simulink model "BuildFlexionExtension2024a"  (R2024a)
settings: Solver=FixedStepAuto  StartTime=0.0  StopTime=inf  FixedStep=1/100  RelTol=1e-3
InitFcn:
  | bp= [0 1 2  5  7  12 16 20 24 28 32 36 40 42 44 46 48 50];
  | spl=[0 3 8 15  25 34 45 60 76 96 110 120 130 138 145 150 155 158]/158;
  | 
  | breakp=[-fliplr(bp(2:end)) bp]*pi/180;
  | spline=[-fliplr(spl(2:end)) spl];
undefined symbols (not defined in the file): Discrete, FSset, Low, qbreak, Time
libraries: arduinolib x34, dspswit3 x11, etargetslib x8, canmsglib x5, dspfdesign x2, ctrlSharedLib x1
settings Model: SimulationMode=external  ExtModeTrigDuration=2  Creator=alexx  LastModifiedBy=roman
settings SolverCC: AutoInsertRateTranBlk=on
settings OptimizationCC: EnhancedBackFolding=on  PassReuseOutputArgsAs=Individual arguments  ZeroExternalMemoryAtStartup=off  ZeroInternalMemoryAtStartup=off  MaxStackSize=64  OptimizeBlockOrder=speed  DifferentSizesBufferReuse=on  OptimizationCustomize=off  EfficientTunableParamExpr=on
settings DebuggingCC: MultiTaskCondExecSysMsg=none  ParameterTunabilityLossMsg=error
settings HardwareCC: ProdBitPerPointer=32  ProdBitPerSizeT=32  ProdBitPerPtrDiffT=32  ProdLargestAtomicInteger=Long  ProdLargestAtomicFloat=Double  ProdWordSize=32  ProdHWDeviceType=ARM Compatible->ARM Cortex  UseEmbeddedCoderFeatures=off  UseSimulinkCoderFeatures=off
settings SFSimCC: MATLABDynamicMemAlloc=off
settings RTWCC: Description=Embedded Coder  SystemTargetFile=ert.tlc  HardwareBoard=Arduino MKR WiFi 1010  TemplateMakefile=ert_default_tmf  Toolchain=Arduino ARM  BuildConfiguration=Faster Runs  GPUComputeCapability=3.5
settings CodeAppCC: ForceParamTrailComments=on  IgnoreCustomStorageClasses=off  OperatorAnnotations=on  SimulinkDataObjDesc=on  SFDataObjDesc=on  InsertBlockDesc=on
settings ERTTargetCC: SupportContinuousTime=on  SupportNonInlinedSFcns=on  SupportVariableSizeSignals=on  ExtModeTransport=3  ExtModeStaticAlloc=on  ExtModeAutomaticAllocSize=off  ExtModeStaticAllocSize=8192  ExtModeMexFile=ext_xcp  ExtModeIntrfLevel=Level2 - Open
settings ConfigComp: CovBoundaryAbsTol=1.0e-5

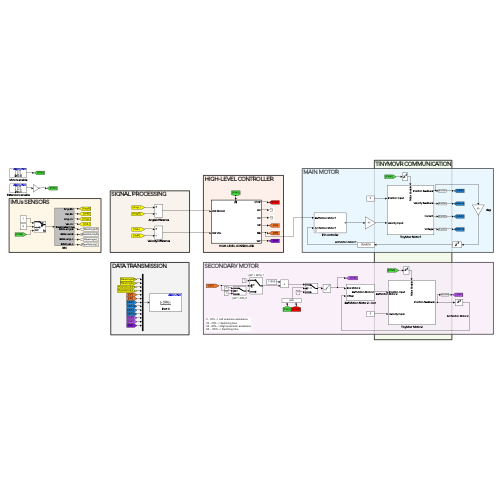
[thumbnail: Simulink's stored preview of the top-level diagram]
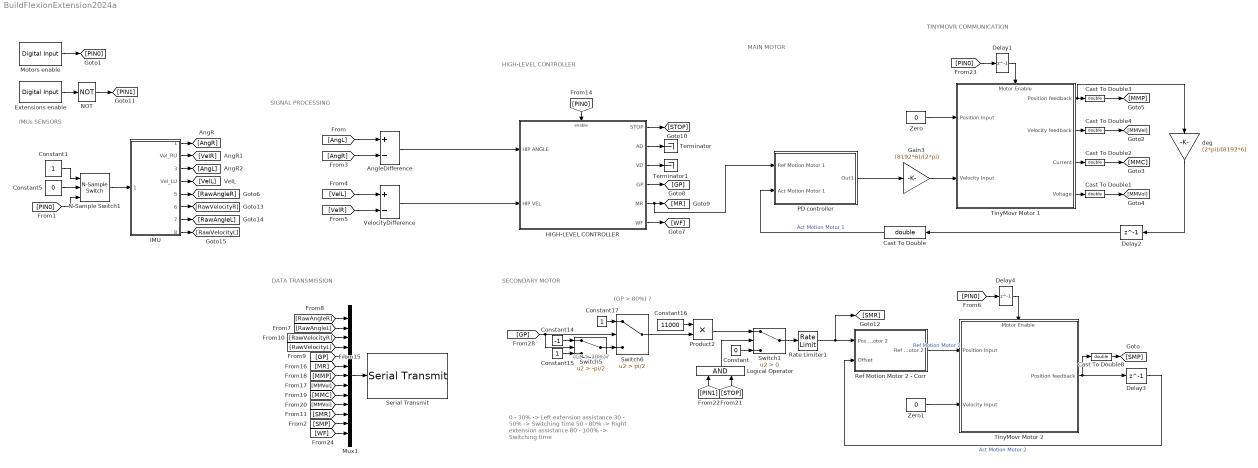
== system BuildFlexionExtension2024a ==
  note: 0 - 30% -> Left extension assistance
      | 30 - 50% -> Switching time
      | 50 - 80% -> Right extension assistance
      | 80 - 100% -> Switching time
  note: (GP > 30%)?
  note: DATA TRANSMISSION
  note: TINYMOVR COMMUNICATION
  note: MAIN MOTOR
  note: SECONDARY MOTOR
  note: HIGH-LEVEL CONTROLLER
  note: SIGNAL PROCESSING
  note: IMUs SENSORS
  note: (GP > 80%) ?
  AngleDifference : Sum  Inputs=+-
  Cast To Double{,1..4,8} (6 alike) : DataTypeConversion  OutDataTypeStr=double  SaturateOnIntegerOverflow=off  RndMeth=Floor
  Constant : Constant  Value=0
  Constant1 : Constant
  Constant14 : Constant  Value=-1
  Constant15 : Constant
  Constant16 : Constant  Value=11000
  Constant17 : Constant
  Constant5 : Constant  Value=0
  Delay{1..4} (4 alike) : Delay  DelayLength=1
  Extensions enable : arduinolib/Digital Input  pinNumber=1  mode=Input Pullup  Direction=input  SampleTime=1/100  blockPlatform=arduino
  Gain3 : Gain  Gain=(8192*6)/(2*pi)  ParamDataTypeStr=single  OutDataTypeStr=single
  HIGH-LEVEL CONTROLLER : Subsystem
  IMU : Subsystem
  Logical Operator : Logic  AllPortsSameDT=off  OutDataTypeStr=boolean
  Motors enable : arduinolib/Digital Input  pinNumber=0  mode=Default  Direction=input  SampleTime=1/100  blockPlatform=arduino
  Mux1 : Mux  Inputs=13
  N-Sample Switch1 : dspswit3/N-Sample Switch  N=10  reset=on  TriggerType=Rising edge  Ts=-1
  NOT : Logic  Operator=NOT  IconShape=distinctive  AllPortsSameDT=off  OutDataTypeStr=boolean
  PD controller : Subsystem  mask{Kp=12, Ki=0, Kd=0.2}
      mask prompts: Kp "P"; Ki "I"; Kd "D"
      mask DialogControl DescGroupVar Prompt: PID Parameters
      mask DialogControl DescTextVar Prompt: Select the values for P I D parameters
  Product2 : Product
  Rate Limiter1 : RateLimiter  RisingSlewLimit=480000  FallingSlewLimit=-480000
  Ref Motion Motor 2 - Corr : Subsystem
  Serial Transmit : arduinolib/Serial Transmit  portNumber=0  sendmode=write  sendformat=Decimal  floatprecision=2  header=[]  terminator=[]  blockPlatform=ARDUINO
  Switch1 : Switch  Criteria=u2 > Threshold  SaturateOnIntegerOverflow=off  InputSameDT=off
  Switch5 : Switch  Criteria=u2 > Threshold  Threshold=-pi/2  SaturateOnIntegerOverflow=off  InputSameDT=off
  Switch6 : Switch  Criteria=u2 > Threshold  Threshold=pi/2  SaturateOnIntegerOverflow=off  InputSameDT=off
  Terminator : Terminator
  Terminator1 : Terminator
  TinyMovr Motor 1 : Subsystem
      settings: PortSchema="{\"entries\":[{\"content\":{\"sides\":[{\"content\":{\"connectorIds\":[\"In1\",\"In2\"]},\"type\":\"ConnectorPlacement.EquallySpacedRectSide\",\"uuid\":\"96eb0664-e7f9-4da5-900f-02ca39bdcd94\"},{\"content\":{\"connectorIds\":[\"Out1\",\"Out2\",\"Out3\",\"Out4\"],\"side\":\"RIGHT\"},\"type\":\"ConnectorPlacement.EquallySpacedRectSide\",\"uuid\":\"3b096aff-b574-48d5-b85c-bddb8debe324\"},{\"content\":{\"connectorIds\":[\"In3\"],\"side\":\"TOP\"},\"type\":\"ConnectorPlacement.EquallySpacedRectSide\",\"uuid\":\"4d311d4a-d713-49d1-a682-ce685fb67b1a\"},{\"content\":{\"side\":\"BOTTOM\"},\"type\":\"ConnectorPlacement.EquallySpacedRectSide\",\"uuid\":\"60a29e50-835b-4a88-8a5f-1647b9a36173\"}]},\"type\":\"ConnectorPlacement.EquallySpacedConnector\",\"uuid\":\"850c9b35-9cb9-4fb8-b21d-22107ea3627a\"}],\"packageUris\":[\"http://schema.mathworks.com/mf0/Connector/R2020b\"],\"version\":\"1.0\"}"
  TinyMovr Motor 2 : Subsystem
      settings: PortSchema="{\"entries\":[{\"content\":{\"sides\":[{\"content\":{\"connectorIds\":[\"In1\",\"In2\"]},\"type\":\"ConnectorPlacement.EquallySpacedRectSide\",\"uuid\":\"96eb0664-e7f9-4da5-900f-02ca39bdcd94\"},{\"content\":{\"connectorIds\":[\"Out1\"],\"side\":\"RIGHT\"},\"type\":\"ConnectorPlacement.EquallySpacedRectSide\",\"uuid\":\"3b096aff-b574-48d5-b85c-bddb8debe324\"},{\"content\":{\"connectorIds\":[\"In3\"],\"side\":\"TOP\"},\"type\":\"ConnectorPlacement.EquallySpacedRectSide\",\"uuid\":\"4d311d4a-d713-49d1-a682-ce685fb67b1a\"}]},\"type\":\"ConnectorPlacement.EquallySpacedConnector\",\"uuid\":\"850c9b35-9cb9-4fb8-b21d-22107ea3627a\"}],\"packageUris\":[\"http://schema.mathworks.com/mf0/Connector/R2020b\"],\"version\":\"1.0\"}"
  VelocityDifference : Sum  Inputs=+-
  Zero : Constant  Value=0  OutDataTypeStr=single
  Zero1 : Constant  Value=0  OutDataTypeStr=single
  deg : Gain  Gain=(2*pi)/(8192*6)  ParamDataTypeStr=single  OutDataTypeStr=single
  wires:
  Cast To Double/1 -> PD controller/2(Act Motion Motor 1)  "Act Motion Motor 1"
  Delay3/1 -> Ref Motion Motor 2 - Corr/2(Offset)  "Act Motion Motor 2"
  TinyMovr Motor 1/1(Position feedback) -> deg/1, Cast To Double3/1
  Ref Motion Motor 2 - Corr/1(Ref Motion Motor 2) -> TinyMovr Motor 2/1(Position Input)  "Ref Motion Motor 2"
  Delay1/1 -> TinyMovr Motor 1/3(Motor Enable)
  Zero/1 -> TinyMovr Motor 1/1(Position Input)
  PD controller/1(Out1) -> Gain3/1
  deg/1 -> Delay2/1
  TinyMovr Motor 2/1(Position feedback) -> Delay3/1, Cast To Double8/1
  Gain3/1 -> TinyMovr Motor 1/2(Velocity Input)
  Rate Limiter1/1 -> Ref Motion Motor 2 - Corr/1(Pos Motor 2), [SMR]
  N-Sample Switch1/1 -> IMU/1(BaselineRemove)
  Constant5/1 -> N-Sample Switch1/2
  Constant1/1 -> N-Sample Switch1/1
  [PIN0] -> N-Sample Switch1/3
  [PIN0] -> HIGH-LEVEL CONTROLLER/Enable
  [PIN0] -> Delay1/1
  HIGH-LEVEL CONTROLLER/5(MR) -> PD controller/1(Ref Motion Motor 1), [MR]
  HIGH-LEVEL CONTROLLER/1(STOP) -> [STOP]
  AngleDifference/1 -> HIGH-LEVEL CONTROLLER/1(HIP ANGLE)
  VelocityDifference/1 -> HIGH-LEVEL CONTROLLER/2(HIP VEL)
  Mux1/1 -> Serial Transmit/1
  [AngL] -> AngleDifference/1
  [AngR] -> AngleDifference/2
  [VelL] -> VelocityDifference/1
  [VelR] -> VelocityDifference/2
  Delay2/1 -> Cast To Double/1
  Zero1/1 -> TinyMovr Motor 2/2(Velocity Input)
  [PIN0] -> Delay4/1
  Delay4/1 -> TinyMovr Motor 2/3(Motor Enable)
  IMU/1(Ang_RU) -> [AngR]
  IMU/2(Vel_RU) -> [VelR]
  IMU/3(Ang_LU) -> [AngL]
  IMU/4(Vel_LU) -> [VelL]
  [RawAngleR] -> Mux1/1
  [RawAngleL] -> Mux1/2
  [RawVelocityR] -> Mux1/3
  [RawVelocityL] -> Mux1/4
  TinyMovr Motor 1/2(Velocity feedback) -> Cast To Double4/1
  TinyMovr Motor 1/3(Current) -> Cast To Double2/1
  TinyMovr Motor 1/4(Voltage) -> Cast To Double1/1
  Cast To Double8/1 -> [SMP]
  [GP] -> Mux1/5
  [MR] -> Mux1/6
  [MMP] -> Mux1/7
  [MMVel] -> Mux1/8
  [MMC] -> Mux1/9
  [MMVol] -> Mux1/10
  Cast To Double1/1 -> [MMVol]
  Cast To Double2/1 -> [MMC]
  Cast To Double4/1 -> [MMVel]
  Cast To Double3/1 -> [MMP]
  HIGH-LEVEL CONTROLLER/2(AD) -> Terminator/1
  HIGH-LEVEL CONTROLLER/3(VD) -> Terminator1/1
  HIGH-LEVEL CONTROLLER/4(GP) -> [GP]
  [STOP] -> Logical Operator/2
  Switch1/1 -> Rate Limiter1/1
  Extensions enable/1 -> NOT/1
  Logical Operator/1 -> Switch1/2
  [PIN1] -> Logical Operator/1
  Constant/1 -> Switch1/3
  NOT/1 -> [PIN1]
  Motors enable/1 -> [PIN0]
  [SMP] -> Mux1/12
  [SMR] -> Mux1/11
  [GP] -> Switch6/2, Switch5/2
  Constant14/1 -> Switch5/1
  Constant15/1 -> Switch5/3
  Constant17/1 -> Switch6/1
  Switch5/1 -> Switch6/3
  Product2/1 -> Switch1/1
  Constant16/1 -> Product2/1
  Switch6/1 -> Product2/2
  HIGH-LEVEL CONTROLLER/6(WF) -> [WF]
  [WF] -> Mux1/13
  IMU/5(RAW_ang_R) -> [RawAngleR]
  IMU/6(RAW_vel_R) -> [RawVelocityR]
  IMU/7(RAW_ang_L) -> [RawAngleL]
  IMU/8(RAW_vel_L) -> [RawVelocityL]

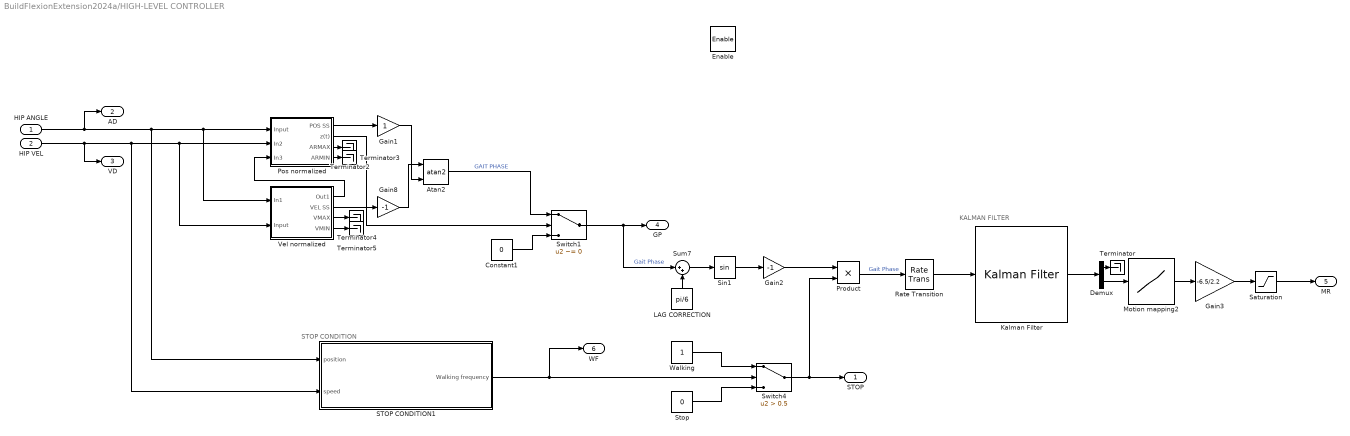
== system BuildFlexionExtension2024a/HIGH-LEVEL CONTROLLER ==
  note: KALMAN FILTER
  note: STOP CONDITION
  HIP ANGLE : Inport
  HIP VEL : Inport  Port=2
  Enable : EnablePort  StatesWhenEnabling=reset
  Atan2 : Trigonometry  Operator=atan2
  Constant1 : Constant  Value=0
  Demux : Demux  Outputs=2
  Gain1 : Gain
  Gain2 : Gain  Gain=-1
  Gain3 : Gain  Gain=-6.5/2.2
  Gain8 : Gain  Gain=-1
  Kalman Filter : ctrlSharedLib/Kalman Filter  TimeDomain=Discrete-Time  UseCurrentEstimator=on  ModelSource=Individual A, B, C, D matrices  ModelSourceVariable=idss  A=[1 0.01;0 1]  B=eye(2)  C=[1 0]  D=zeros(2)  NumberOfStates=1  NumberOfInputs=1  NumberOfOutputs=1  InitialEstimateSource=Dialog  X0=0  P0=10  UseK=off  UseGH=off  NumberOfProcessNoiseInputs=2  G=1  TimeInvariantG=on  H=0  TimeInvariantH=on  Q=0.02  TimeInvariantQ=on  R=0.75  TimeInvariantR=on  N=0  TimeInvariantN=on  AddInputPort=off  AddEnablePort=off  OutputEstimatedY=off  OutputP=off  Ts=-1
  LAG CORRECTION : Constant  Value=pi/6
  Motion mapping2 : Lookup_n-D  NumberOfTableDimensions=1  BreakpointsForDimension1=breakp  BreakpointsForDimension2=qbreak(:,2)  Table=spline  InterpMethod=Cubic spline  ExtrapMethod=Cubic spline  InternalRulePriority=Speed  RndMeth=Simplest
  Pos normalized : Subsystem
  Product : Product
  Rate Transition : RateTransition  OutPortSampleTime=0.01
  STOP CONDITION1 : Subsystem
  Saturation : Saturate  UpperLimit=600*pi/180  LowerLimit=-600*pi/180
  Sin1 : Trigonometry
  Stop : Constant  Value=0
  Sum7 : Sum  Inputs=|++
  Switch1 : Switch  Criteria=u2 ~= 0  SaturateOnIntegerOverflow=off  InputSameDT=off
  Switch4 : Switch  Criteria=u2 > Threshold  Threshold=0.5  SaturateOnIntegerOverflow=off  InputSameDT=off
  Terminator{,2..5} (5 alike) : Terminator
  Vel normalized : Subsystem
  Walking : Constant
  STOP : Outport
  AD : Outport  Port=2
  VD : Outport  Port=3
  GP : Outport  Port=4
  MR : Outport  Port=5
  WF : Outport  Port=6
  wires:
  Kalman Filter/1 -> Demux/1
  Gain8/1 -> Atan2/1
  Gain2/1 -> Product/1
  Gain3/1 -> Saturation/1
  Rate Transition/1 -> Kalman Filter/1
  Atan2/1 -> Switch1/1  "GAIT PHASE"
  Sin1/1 -> Gain2/1
  Switch1/1 -> GP/1, Sum7/1  "Gait Phase"
  Product/1 -> Rate Transition/1  "Gait Phase"
  Constant1/1 -> Switch1/3
  Motion mapping2/1 -> Gain3/1
  Demux/1 -> Terminator/1
  LAG CORRECTION/1 -> Sum7/2
  Gain1/1 -> Atan2/2
  Saturation/1 -> MR/1
  Pos normalized/1(POS SS) -> Gain1/1
  Pos normalized/2(z(t)) -> Switch1/2
  Vel normalized/1(Out1) -> Pos normalized/3(In3)
  Vel normalized/2(VEL SS) -> Gain8/1
  Pos normalized/3(ARMAX) -> Terminator2/1
  Pos normalized/4(ARMIN) -> Terminator3/1
  Vel normalized/3(VMAX) -> Terminator4/1
  Vel normalized/4(VMIN) -> Terminator5/1
  Sum7/1 -> Sin1/1
  Demux/2 -> Motion mapping2/1
  Walking/1 -> Switch4/1
  HIP VEL/1 -> VD/1, STOP CONDITION1/2(speed), Vel normalized/2(Input), Pos normalized/2(In2)
  Switch4/1 -> STOP/1, Product/2
  Stop/1 -> Switch4/3
  STOP CONDITION1/1(Walking frequency) -> WF/1, Switch4/2
  HIP ANGLE/1 -> STOP CONDITION1/1(position), Vel normalized/1(In1), Pos normalized/1(Input), AD/1

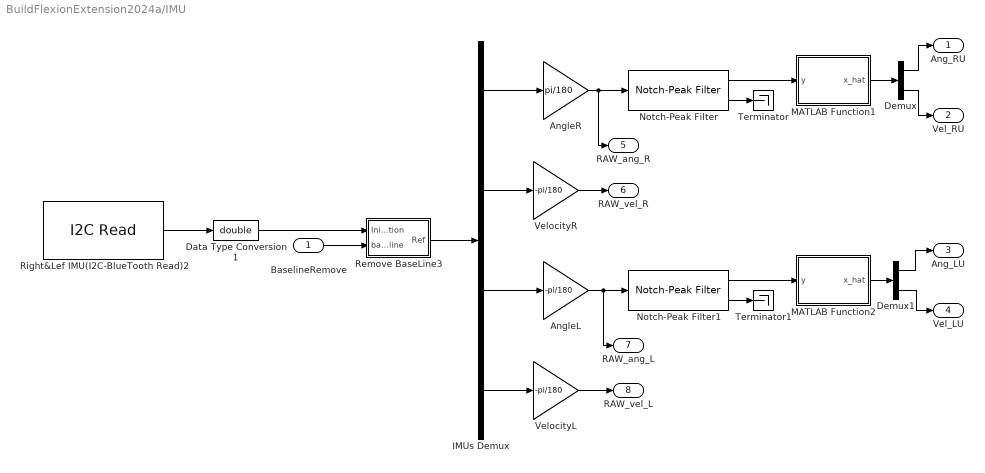
== system BuildFlexionExtension2024a/IMU ==
  BaselineRemove : Inport
  AngleL : Gain  Gain=-pi/180
  AngleR : Gain  Gain=pi/180
  Data Type Conversion1 : DataTypeConversion  OutDataTypeStr=double  SaturateOnIntegerOverflow=off  RndMeth=Floor
  Demux : Demux  Outputs=2
  Demux1 : Demux  Outputs=2
  IMUs Demux : Demux
  MATLAB Function1 : MATLAB Function  TreatAsAtomicUnit=on
  MATLAB Function2 : MATLAB Function  TreatAsAtomicUnit=on
  Notch-Peak Filter : dspfdesign/Notch-Peak Filter  Specification=Bandwidth and center frequency  BandwidthPort=off  Bandwidth=0.1  QualityFactorPort=off  QualityFactor=5  CenterFrequencyPort=off  CenterFrequency=0  BandwidthCoefficientPort=off  BandwidthCoefficient=0.72654  CenterFrequencyCoefficientPort=off  CenterFrequencyCoefficient=0  Output=Notch and Peak  SampleRateMode=Specify on dialog  SampleRate=100  SimulateUsing=Code generation
  Notch-Peak Filter1 : dspfdesign/Notch-Peak Filter  Specification=Bandwidth and center frequency  BandwidthPort=off  Bandwidth=0.1  QualityFactorPort=off  QualityFactor=5  CenterFrequencyPort=off  CenterFrequency=0  BandwidthCoefficientPort=off  BandwidthCoefficient=0.72654  CenterFrequencyCoefficientPort=off  CenterFrequencyCoefficient=0  Output=Notch and Peak  SampleRateMode=Specify on dialog  SampleRate=100  SimulateUsing=Code generation
  Remove BaseLine3 : Subsystem
  Right&Lef IMU(I2C-BlueTooth Read)2 : arduinolib/I2C Read  I2CModule=0  Mode=Master  SlaveAddress=45  SlaveByteOrder=LittleEndian  Direction=Receiver  RegisterAddressMode=off  RegisterAddress=0  SlaveDataType=single  DataLength=4  NoAck=off  RepeatedStart=off  OutputStatus=off  blockPlatform=ARDUINO  SampleTime=0.01
  Terminator : Terminator
  Terminator1 : Terminator
  VelocityL : Gain  Gain=-pi/180
  VelocityR : Gain  Gain=-pi/180
  Ang_RU : Outport
  Vel_RU : Outport  Port=2
  Ang_LU : Outport  Port=3
  Vel_LU : Outport  Port=4
  RAW_ang_R : Outport  Port=5
  RAW_vel_R : Outport  Port=6
  RAW_ang_L : Outport  Port=7
  RAW_vel_L : Outport  Port=8
  wires:
  BaselineRemove/1 -> Remove BaseLine3/2(baseline)
  Data Type Conversion1/1 -> Remove BaseLine3/1(Initial Motion)
  Right&Lef IMU(I2C-BlueTooth Read)2/1 -> Data Type Conversion1/1
  Remove BaseLine3/1(Ref) -> IMUs Demux/1
  IMUs Demux/2 -> VelocityR/1
  IMUs Demux/1 -> AngleR/1
  AngleR/1 -> RAW_ang_R/1, Notch-Peak Filter/1
  IMUs Demux/3 -> AngleL/1
  IMUs Demux/4 -> VelocityL/1
  AngleL/1 -> RAW_ang_L/1, Notch-Peak Filter1/1
  Notch-Peak Filter/1 -> MATLAB Function1/1(y)
  Notch-Peak Filter/2 -> Terminator/1
  Notch-Peak Filter1/1 -> MATLAB Function2/1(y)
  Notch-Peak Filter1/2 -> Terminator1/1
  MATLAB Function1/1(x_hat) -> Demux/1
  Demux/1 -> Ang_RU/1
  Demux/2 -> Vel_RU/1
  MATLAB Function2/1(x_hat) -> Demux1/1
  Demux1/1 -> Ang_LU/1
  Demux1/2 -> Vel_LU/1
  VelocityR/1 -> RAW_vel_R/1
  VelocityL/1 -> RAW_vel_L/1

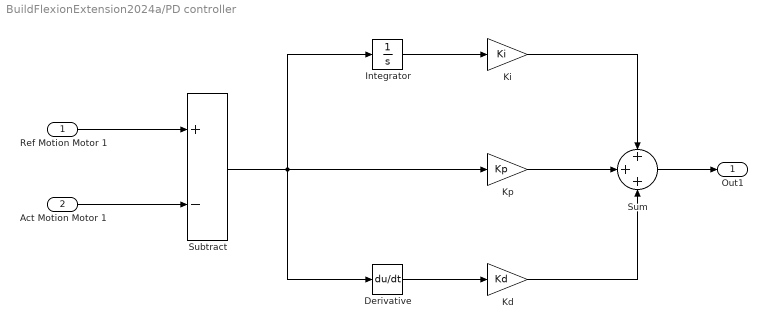
== system BuildFlexionExtension2024a/PD controller ==
  Ref Motion Motor 1 : Inport
  Act Motion Motor 1 : Inport  Port=2
  Derivative : Derivative
  Integrator : Integrator
  Kd : Gain  Gain=Kd
  Ki : Gain  Gain=Ki
  Kp : Gain  Gain=Kp
  Subtract : Sum  Inputs=+-
  Sum : Sum  Inputs=+++
  Out1 : Outport
  wires:
  Act Motion Motor 1/1 -> Subtract/2
  Ref Motion Motor 1/1 -> Subtract/1
  Integrator/1 -> Ki/1
  Sum/1 -> Out1/1
  Ki/1 -> Sum/1
  Kp/1 -> Sum/2
  Kd/1 -> Sum/3
  Subtract/1 -> Derivative/1, Kp/1, Integrator/1
  Derivative/1 -> Kd/1

== system BuildFlexionExtension2024a/Ref Motion Motor 2 - Corr ==
  note: The blocks are making sure the motor’s commanded motion is always consistent with its measured position. If the encoder hasn’t moved (maybe at power-up or during a pause), the system falls back to an offset value. The sum block then adjusts the commanded trajectory by this alignment term, so the reference sent to the motor matches reality.
  Pos Motor 2 : Inport
  Offset : Inport  Port=2
  Add : Sum
  Constant : Constant  Value=0
  Delay : Delay  DelayLength=1
  Delay1 : Delay  DelayLength=1
  Switch1 : Switch  Criteria=u2 ~= 0  SaturateOnIntegerOverflow=off  InputSameDT=off
  Ref Motion Motor 2 : Outport
  wires:
  Offset/1 -> Delay1/1  "Motor Encoder [rad]"
  Delay1/1 -> Switch1/2
  Switch1/1 -> Delay/1, Add/2
  Delay/1 -> Switch1/1
  Add/1 -> Ref Motion Motor 2/1
  Pos Motor 2/1 -> Add/1
  Constant/1 -> Switch1/3

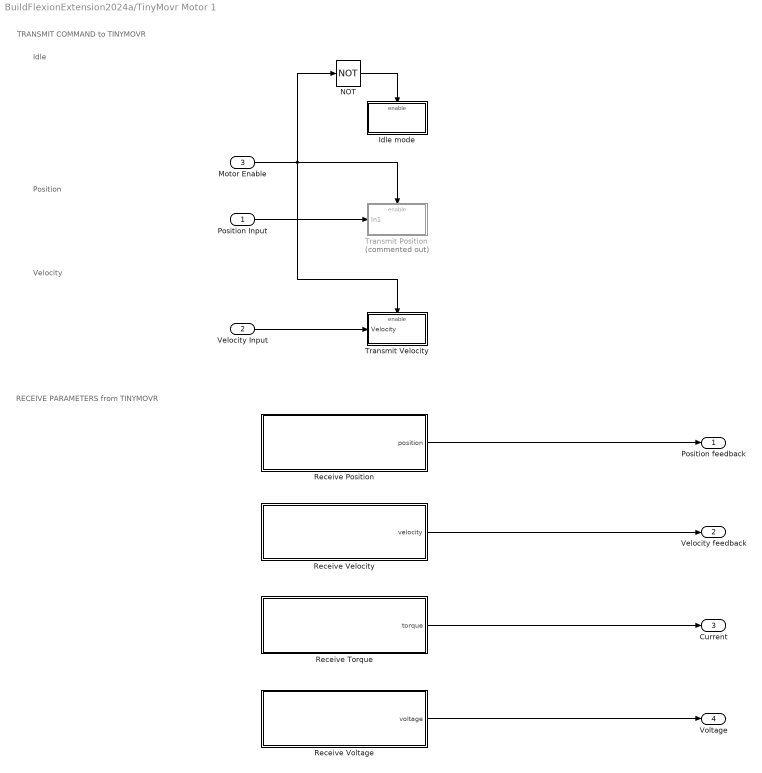
== system BuildFlexionExtension2024a/TinyMovr Motor 1 ==
  note: Idle
  note: Velocity
  note: TRANSMIT COMMAND to TINYMOVR
  note: Position
  note: RECEIVE PARAMETERS from TINYMOVR
  Position Input : Inport
  Velocity Input : Inport  Port=2
  Motor Enable : Inport  Port=3
  Idle mode : Subsystem  TreatAsAtomicUnit=on
  NOT : Logic  Operator=NOT  AllPortsSameDT=off  OutDataTypeStr=boolean
  Receive Position : Subsystem
  Receive Torque : Subsystem
  Receive Velocity : Subsystem
  Receive Voltage : Subsystem
  Transmit Position : Subsystem  Commented=on  TreatAsAtomicUnit=on
  Transmit Velocity : Subsystem  TreatAsAtomicUnit=on
  Position feedback : Outport
  Velocity feedback : Outport  Port=2
  Current : Outport  Port=3
  Voltage : Outport  Port=4
  wires:
  Position Input/1 -> Transmit Position/1(In1)
  NOT/1 -> Idle mode/Enable
  Motor Enable/1 -> Transmit Position/Enable, Transmit Velocity/Enable, NOT/1
  Velocity Input/1 -> Transmit Velocity/1(Velocity)
  Receive Position/1(position) -> Position feedback/1
  Receive Velocity/1(velocity) -> Velocity feedback/1
  Receive Torque/1(torque) -> Current/1
  Receive Voltage/1(voltage) -> Voltage/1

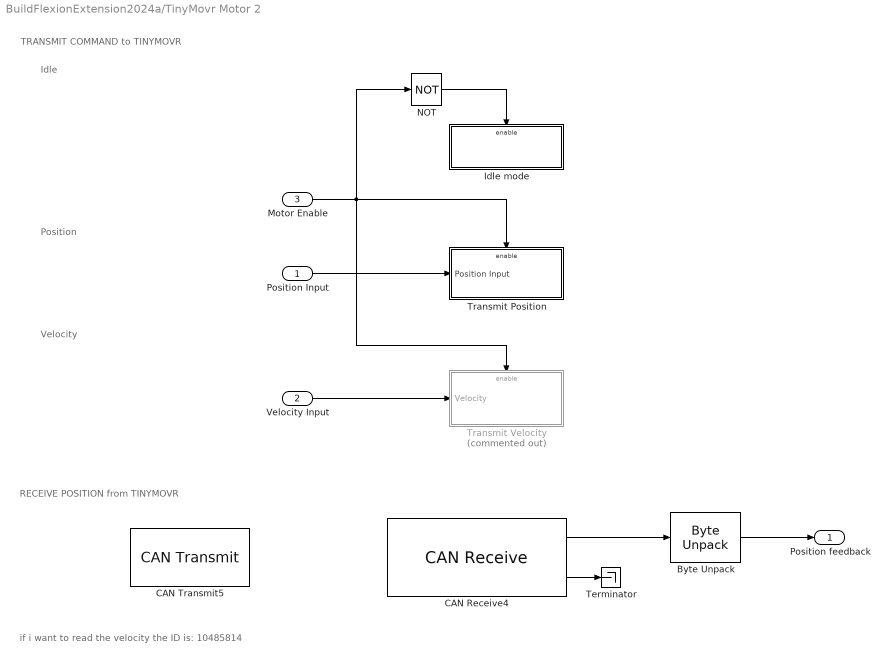
== system BuildFlexionExtension2024a/TinyMovr Motor 2 ==
  note: if i want to read the velocity the ID is: 10485814
  note: Idle
  note: Velocity
  note: TRANSMIT COMMAND to TINYMOVR
  note: RECEIVE POSITION from TINYMOVR
  note: Position
  Position Input : Inport
  Velocity Input : Inport  Port=2
  Motor Enable : Inport  Port=3
  Byte Unpack : etargetslib/Byte Unpack  dimensions={[1]}  datatypes={'single'}  byteAlign=1
      settings: LibrarySourceBlock=embeddedtargetslib/Host Communication/Byte Unpack
  CAN Receive4 : arduinolib/CAN Receive  outputDataType=Raw data  identifierType=Extended (29-bit identifier)  messageId=4194359  msgLength=4  SampleTime=0.01  outputError=off  outputRemote=off
  CAN Transmit5 : arduinolib/CAN Transmit  inputDataType=Raw data  BlockingMode_=off  BlockTimeout_=1  outputStatus=off  identifierType=Extended (29-bit identifier)  messageId=4194359  msgLength=0  remoteFrame=on
  Idle mode : Subsystem  TreatAsAtomicUnit=on
  NOT : Logic  Operator=NOT  AllPortsSameDT=off  OutDataTypeStr=boolean
  Terminator : Terminator
  Transmit Position : Subsystem  TreatAsAtomicUnit=on
  Transmit Velocity : Subsystem  Commented=on  TreatAsAtomicUnit=on
  Position feedback : Outport
  wires:
  CAN Receive4/1 -> Byte Unpack/1
  CAN Receive4/2 -> Terminator/1
  Byte Unpack/1 -> Position feedback/1
  Position Input/1 -> Transmit Position/1(Position Input)
  NOT/1 -> Idle mode/Enable
  Velocity Input/1 -> Transmit Velocity/1(Velocity)
  Motor Enable/1 -> Transmit Position/Enable, Transmit Velocity/Enable, NOT/1

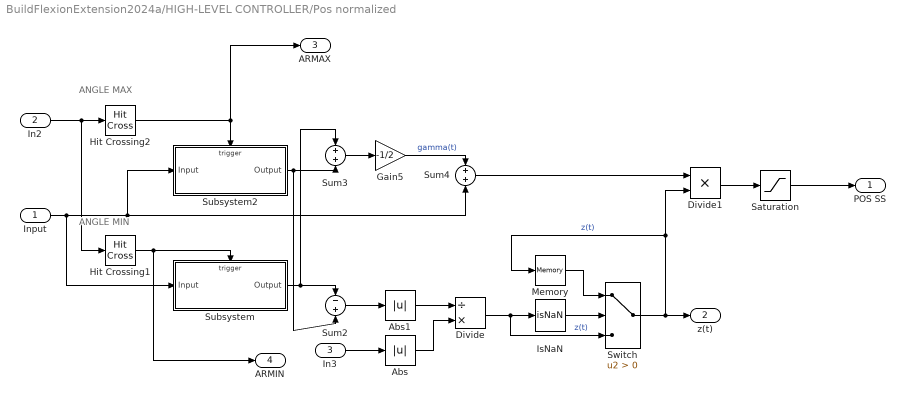
== system BuildFlexionExtension2024a/HIGH-LEVEL CONTROLLER/Pos normalized ==
  note: ANGLE MIN
  note: ANGLE MAX
  Input : Inport
  In2 : Inport  Port=2
  In3 : Inport  Port=3
  Abs : Abs  SaturateOnIntegerOverflow=off
  Abs1 : Abs  SaturateOnIntegerOverflow=off
  Divide : Product  Inputs=/*
  Divide1 : Product  Inputs=**
  Gain5 : Gain  Gain=-1/2
  Hit Crossing1 : HitCross  HitCrossingOffset=-1  HitCrossingDirection=rising
  Hit Crossing2 : HitCross  HitCrossingOffset=1  HitCrossingDirection=falling
  IsNaN : RelationalOperator  Operator=isNaN  OutDataTypeStr=boolean  RndMeth=Simplest  InputSameDT=off
  Memory : Memory
  Saturation : Saturate  UpperLimit=10  LowerLimit=-10
  Subsystem : Subsystem
  Subsystem2 : Subsystem
  Sum2 : Sum  Inputs=-+
  Sum3 : Sum
  Sum4 : Sum
  Switch : Switch  Criteria=u2 > Threshold  SaturateOnIntegerOverflow=off  InputSameDT=off
  POS SS : Outport
  z(t) : Outport  Port=2
  ARMAX : Outport  Port=3
  ARMIN : Outport  Port=4
  wires:
  Hit Crossing2/1 -> Subsystem2/Trigger, ARMAX/1
  Subsystem2/1(Output) -> Sum3/2, Sum2/2
  Sum4/1 -> Divide1/1
  Sum3/1 -> Gain5/1
  Subsystem/1(Output) -> Sum2/1, Sum3/1
  Hit Crossing1/1 -> ARMIN/1, Subsystem/Trigger
  Input/1 -> Subsystem2/1(Input), Sum4/2, Subsystem/1(Input)
  In2/1 -> Hit Crossing1/1, Hit Crossing2/1
  Sum2/1 -> Abs1/1
  In3/1 -> Abs/1
  Gain5/1 -> Sum4/1  "gamma(t)"
  Abs1/1 -> Divide/1
  Abs/1 -> Divide/2
  Divide/1 -> IsNaN/1, Switch/3  "z(t)"
  Memory/1 -> Switch/1
  IsNaN/1 -> Switch/2
  Switch/1 -> Memory/1, Divide1/2, z(t)/1  "z(t)"
  Divide1/1 -> Saturation/1
  Saturation/1 -> POS SS/1

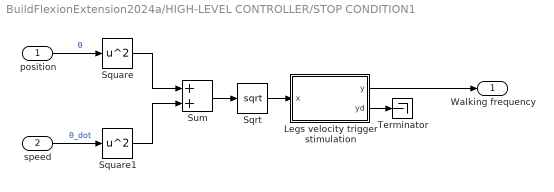
== system BuildFlexionExtension2024a/HIGH-LEVEL CONTROLLER/STOP CONDITION1 ==
  position : Inport
  speed : Inport  Port=2
  Legs velocity trigger stimulation : Subsystem  mask{wn=20, zt=1, x0=0}
      mask prompts: wn "Cut-off frequency (rad/s)"; zt "Damping ratio"; x0 "Initial Condition"
      mask Display: disp('Second-Order\nLow-Pass Filter');
  Sqrt : Sqrt
  Square : Math  Operator=square
  Square1 : Math  Operator=square
  Sum : Sum
  Terminator : Terminator
  Walking frequency : Outport
  wires:
  position/1 -> Square/1  "θ"
  speed/1 -> Square1/1  "θ_dot"
  Square/1 -> Sum/1
  Square1/1 -> Sum/2
  Sum/1 -> Sqrt/1
  Sqrt/1 -> Legs velocity trigger stimulation/1(x)
  Legs velocity trigger stimulation/1(y) -> Walking frequency/1
  Legs velocity trigger stimulation/2(yd) -> Terminator/1

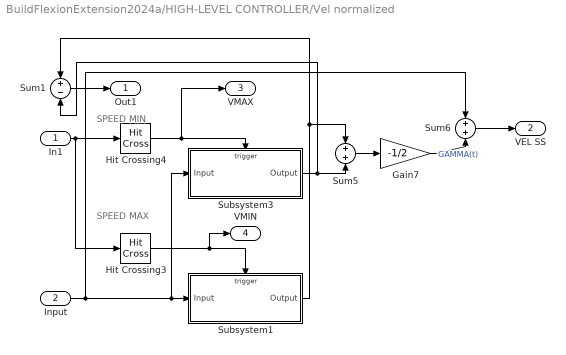
== system BuildFlexionExtension2024a/HIGH-LEVEL CONTROLLER/Vel normalized ==
  note: SPEED MAX
  note: SPEED MIN
  In1 : Inport
  Input : Inport  Port=2
  Gain7 : Gain  Gain=-1/2
  Hit Crossing3 : HitCross  HitCrossingOffset=-0.1  HitCrossingDirection=rising
  Hit Crossing4 : HitCross  HitCrossingOffset=0.1  HitCrossingDirection=falling
  Subsystem1 : Subsystem
  Subsystem3 : Subsystem
  Sum1 : Sum  Inputs=+-
  Sum5 : Sum
  Sum6 : Sum
  Out1 : Outport
  VEL SS : Outport  Port=2
  VMAX : Outport  Port=3
  VMIN : Outport  Port=4
  wires:
  Sum5/1 -> Gain7/1
  Subsystem1/1(Output) -> Sum1/1, Sum5/1
  Sum1/1 -> Out1/1
  Subsystem3/1(Output) -> Sum1/2, Sum5/2
  In1/1 -> Hit Crossing4/1, Hit Crossing3/1
  Gain7/1 -> Sum6/2  "GAMMA(t)"
  Sum6/1 -> VEL SS/1
  Input/1 -> Sum6/1, Subsystem1/1(Input), Subsystem3/1(Input)
  Hit Crossing3/1 -> VMIN/1, Subsystem1/Trigger
  Hit Crossing4/1 -> VMAX/1, Subsystem3/Trigger

== system BuildFlexionExtension2024a/IMU/Remove BaseLine3 ==
  note: Subsystem2
  Initial Motion : Inport
  baseline : Inport  Port=2
  Delay : Delay
  Memory1 : Memory
  Sum9 : Sum  Inputs=|+-
  Switch1 : Switch  Criteria=u2 > Threshold  SaturateOnIntegerOverflow=off  InputSameDT=off
  Ref : Outport
  wires:
  Sum9/1 -> Ref/1
  Switch1/1 -> Delay/1, Sum9/2
  Delay/1 -> Memory1/1
  Initial Motion/1 -> Switch1/1, Sum9/1
  baseline/1 -> Switch1/2
  Memory1/1 -> Switch1/3

== system BuildFlexionExtension2024a/TinyMovr Motor 1/Idle mode ==
  Enable : EnablePort
  CAN Transmit1 : arduinolib/CAN Transmit  inputDataType=Raw data  BlockingMode_=off  BlockTimeout_=1  outputStatus=off  identifierType=Extended (29-bit identifier)  messageId=2097192  msgLength=0  remoteFrame=off

== system BuildFlexionExtension2024a/TinyMovr Motor 1/Receive Position ==
  Byte Unpack : etargetslib/Byte Unpack  dimensions={[1]}  datatypes={'single'}  byteAlign=1
      settings: LibrarySourceBlock=embeddedtargetslib/Host Communication/Byte Unpack
  CAN Receive : arduinolib/CAN Receive  outputDataType=Raw data  identifierType=Extended (29-bit identifier)  messageId=2097207  msgLength=4  SampleTime=1/100  outputError=off  outputRemote=off
  CAN Transmit3 : arduinolib/CAN Transmit  inputDataType=Raw data  BlockingMode_=off  BlockTimeout_=1  outputStatus=off  identifierType=Extended (29-bit identifier)  messageId=2097207  msgLength=0  remoteFrame=on
  Terminator : Terminator
  position : Outport
  wires:
  CAN Receive/2 -> Terminator/1
  CAN Receive/1 -> Byte Unpack/1
  Byte Unpack/1 -> position/1

== system BuildFlexionExtension2024a/TinyMovr Motor 1/Receive Torque ==
  Byte Unpack : etargetslib/Byte Unpack  dimensions={[1]}  datatypes={'single'}  byteAlign=1
      settings: LibrarySourceBlock=embeddedtargetslib/Host Communication/Byte Unpack
  CAN Receive : arduinolib/CAN Receive  outputDataType=Raw data  identifierType=Extended (29-bit identifier)  messageId=2097185  msgLength=4  SampleTime=0.01  outputError=off  outputRemote=off
  CAN Transmit3 : arduinolib/CAN Transmit  inputDataType=Raw data  BlockingMode_=off  BlockTimeout_=1  outputStatus=off  identifierType=Extended (29-bit identifier)  messageId=2097185  msgLength=0  remoteFrame=on
  Terminator : Terminator
  torque : Outport
  wires:
  CAN Receive/1 -> Byte Unpack/1
  CAN Receive/2 -> Terminator/1
  Byte Unpack/1 -> torque/1

== system BuildFlexionExtension2024a/TinyMovr Motor 1/Receive Velocity ==
  Byte Unpack : etargetslib/Byte Unpack  dimensions={[1]}  datatypes={'single'}  byteAlign=1
      settings: LibrarySourceBlock=embeddedtargetslib/Host Communication/Byte Unpack
  CAN Receive : arduinolib/CAN Receive  outputDataType=Raw data  identifierType=Extended (29-bit identifier)  messageId=2097208  msgLength=4  SampleTime=1/100  outputError=off  outputRemote=off
  CAN Transmit3 : arduinolib/CAN Transmit  inputDataType=Raw data  BlockingMode_=off  BlockTimeout_=1  outputStatus=off  identifierType=Extended (29-bit identifier)  messageId=2097208  msgLength=0  remoteFrame=on
  Terminator : Terminator
  velocity : Outport
  wires:
  Byte Unpack/1 -> velocity/1
  CAN Receive/2 -> Terminator/1
  CAN Receive/1 -> Byte Unpack/1

== system BuildFlexionExtension2024a/TinyMovr Motor 1/Receive Voltage ==
  Byte Unpack : etargetslib/Byte Unpack  dimensions={[1]}  datatypes={'single'}  byteAlign=1
      settings: LibrarySourceBlock=embeddedtargetslib/Host Communication/Byte Unpack
  CAN Receive : arduinolib/CAN Receive  outputDataType=Raw data  identifierType=Extended (29-bit identifier)  messageId=2097156  msgLength=4  SampleTime=0.01  outputError=off  outputRemote=off
  CAN Transmit3 : arduinolib/CAN Transmit  inputDataType=Raw data  BlockingMode_=off  BlockTimeout_=1  outputStatus=off  identifierType=Extended (29-bit identifier)  messageId=2097156  msgLength=0  remoteFrame=on
  Terminator : Terminator
  voltage : Outport
  wires:
  CAN Receive/1 -> Byte Unpack/1
  CAN Receive/2 -> Terminator/1
  Byte Unpack/1 -> voltage/1

== system BuildFlexionExtension2024a/TinyMovr Motor 1/Transmit Position ==
  In1 : Inport
  Enable : EnablePort
  N-Sample Enable : dspswit3/N-Sample Enable  N=5  ActiveLevel=Low (0)  reset=off  TriggerType=Rising edge  Ts=1/100  DataType=Logical
      settings: LibrarySourceBlock=|
      | dspsrcs4/N-Sample
      | Enable
  NOT : Logic  Operator=NOT  IconShape=distinctive  AllPortsSameDT=off  OutDataTypeStr=boolean
  Subsystem : Subsystem
  Subsystem1 : Subsystem
  wires:
  N-Sample Enable/1 -> Subsystem/Enable, NOT/1
  Subsystem/1(Out1) -> Subsystem1/1(" ")
  In1/1 -> Subsystem1/2(In1)
  NOT/1 -> Subsystem1/Enable

== system BuildFlexionExtension2024a/TinyMovr Motor 1/Transmit Velocity ==
  Velocity : Inport
  Enable : EnablePort
  N-Sample Enable : dspswit3/N-Sample Enable  N=5  ActiveLevel=Low (0)  reset=off  TriggerType=Rising edge  Ts=1/100  DataType=Logical
      settings: LibrarySourceBlock=|
      | dspsrcs4/N-Sample
      | Enable
  NOT : Logic  Operator=NOT  IconShape=distinctive  AllPortsSameDT=off  OutDataTypeStr=boolean
  Subsystem : Subsystem
  Subsystem1 : Subsystem
  wires:
  N-Sample Enable/1 -> Subsystem/Enable, NOT/1
  Velocity/1 -> Subsystem1/1(Velocity)
  NOT/1 -> Subsystem1/Enable

== system BuildFlexionExtension2024a/TinyMovr Motor 2/Idle mode ==
  Enable : EnablePort
  CAN Transmit1 : arduinolib/CAN Transmit  inputDataType=Raw data  BlockingMode_=off  BlockTimeout_=1  outputStatus=off  identifierType=Extended (29-bit identifier)  messageId=10485797  msgLength=0  remoteFrame=off

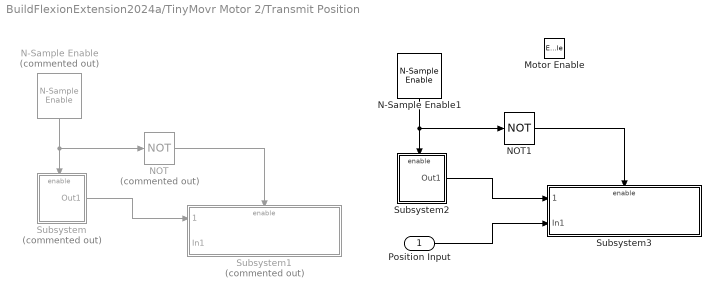
== system BuildFlexionExtension2024a/TinyMovr Motor 2/Transmit Position ==
  Position Input : Inport
  Motor Enable : EnablePort
  N-Sample Enable : dspswit3/N-Sample Enable  Commented=on  N=5  ActiveLevel=Low (0)  reset=off  TriggerType=Rising edge  Ts=1/FSset  DataType=Logical
      settings: LibrarySourceBlock=|
      | dspsrcs4/N-Sample
      | Enable
  N-Sample Enable1 : dspswit3/N-Sample Enable  N=5  ActiveLevel=Low (0)  reset=off  TriggerType=Rising edge  Ts=1/100  DataType=Logical
  NOT : Logic  Commented=on  Operator=NOT  IconShape=distinctive  AllPortsSameDT=off  OutDataTypeStr=boolean
  NOT1 : Logic  Operator=NOT  IconShape=distinctive  AllPortsSameDT=off  OutDataTypeStr=boolean
  Subsystem : Subsystem  Commented=on
  Subsystem1 : Subsystem  Commented=on
  Subsystem2 : Subsystem
  Subsystem3 : Subsystem
  wires:
  N-Sample Enable/1 -> Subsystem/Enable, NOT/1
  Subsystem/1(Out1) -> Subsystem1/1(" ")
  NOT/1 -> Subsystem1/Enable
  Subsystem2/1(Out1) -> Subsystem3/1(" ")
  N-Sample Enable1/1 -> Subsystem2/Enable, NOT1/1
  NOT1/1 -> Subsystem3/Enable
  Position Input/1 -> Subsystem3/2(In1)

== system BuildFlexionExtension2024a/TinyMovr Motor 2/Transmit Velocity ==
  Velocity : Inport
  Enable : EnablePort
  N-Sample Enable : dspswit3/N-Sample Enable  N=5  ActiveLevel=Low (0)  reset=off  TriggerType=Rising edge  Ts=1/FSset  DataType=Logical
      settings: LibrarySourceBlock=|
      | dspsrcs4/N-Sample
      | Enable
  NOT : Logic  Operator=NOT  IconShape=distinctive  AllPortsSameDT=off  OutDataTypeStr=boolean
  Subsystem : Subsystem
  Subsystem1 : Subsystem
  wires:
  N-Sample Enable/1 -> Subsystem/Enable, NOT/1
  Velocity/1 -> Subsystem1/1(Velocity)
  NOT/1 -> Subsystem1/Enable

== system BuildFlexionExtension2024a/HIGH-LEVEL CONTROLLER/Pos normalized/Subsystem ==
  Input : Inport
  Trigger : TriggerPort  VariantControl=Variant  PortDimensions=1
  Output : Outport
  wires:
  Input/1 -> Output/1

== system BuildFlexionExtension2024a/HIGH-LEVEL CONTROLLER/Pos normalized/Subsystem2 ==
  Input : Inport
  Trigger : TriggerPort  VariantControl=Variant  PortDimensions=1
  Output : Outport
  wires:
  Input/1 -> Output/1

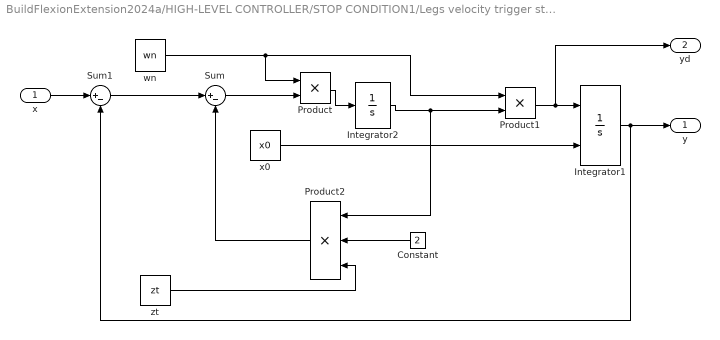
== system BuildFlexionExtension2024a/HIGH-LEVEL CONTROLLER/STOP CONDITION1/Legs velocity trigger stimulation ==
  x : Inport
  Constant : Constant  Value=2
  Integrator1 : Integrator  InitialConditionSource=external
  Integrator2 : Integrator
  Product : Product  RndMeth=Zero
  Product1 : Product  RndMeth=Zero
  Product2 : Product  Inputs=3  RndMeth=Zero
  Sum : Sum  Inputs=|+-
  Sum1 : Sum  Inputs=|+-
  wn : Constant  Value=wn
  x0 : Constant  Value=x0
  zt : Constant  Value=zt
  y : Outport  VectorParamsAs1DForOutWhenUnconnected=off
  yd : Outport  Port=2  VectorParamsAs1DForOutWhenUnconnected=off
  wires:
  Sum/1 -> Product/2
  wn/1 -> Product/1, Product1/1
  Sum1/1 -> Sum/1
  x0/1 -> Integrator1/2
  Integrator2/1 -> Product1/2, Product2/1
  Product/1 -> Integrator2/1
  x/1 -> Sum1/1
  Product1/1 -> Integrator1/1, yd/1
  Integrator1/1 -> Sum1/2, y/1
  Product2/1 -> Sum/2
  zt/1 -> Product2/3
  Constant/1 -> Product2/2

== system BuildFlexionExtension2024a/HIGH-LEVEL CONTROLLER/Vel normalized/Subsystem1 ==
  Input : Inport
  Trigger : TriggerPort  VariantControl=Variant  PortDimensions=1
  Output : Outport
  wires:
  Input/1 -> Output/1

== system BuildFlexionExtension2024a/HIGH-LEVEL CONTROLLER/Vel normalized/Subsystem3 ==
  Input : Inport
  Trigger : TriggerPort  VariantControl=Variant  PortDimensions=1
  Output : Outport
  wires:
  Input/1 -> Output/1

== system BuildFlexionExtension2024a/TinyMovr Motor 1/Transmit Position/Subsystem ==
  Enable : EnablePort
  Byte Unpack : etargetslib/Byte Unpack  dimensions={[1]}  datatypes={'single'}  byteAlign=1
      settings: LibrarySourceBlock=embeddedtargetslib/Host Communication/Byte Unpack
  CAN Receive : arduinolib/CAN Receive  outputDataType=Raw data  identifierType=Extended (29-bit identifier)  messageId=2097207  msgLength=4  SampleTime=1/100  outputError=off  outputRemote=off
  CAN Transmit3 : arduinolib/CAN Transmit  inputDataType=Raw data  BlockingMode_=off  BlockTimeout_=1  outputStatus=off  identifierType=Extended (29-bit identifier)  messageId=2097207  msgLength=0  remoteFrame=on
  Terminator : Terminator
  Out1 : Outport
  wires:
  CAN Receive/2 -> Terminator/1
  CAN Receive/1 -> Byte Unpack/1
  Byte Unpack/1 -> Out1/1

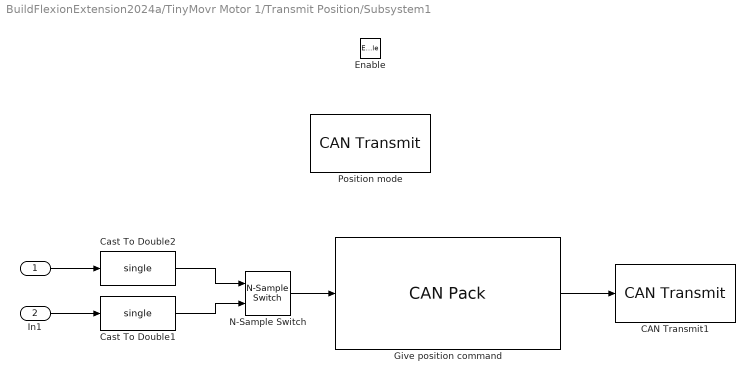
== system BuildFlexionExtension2024a/TinyMovr Motor 1/Transmit Position/Subsystem1 ==
  " " : Inport
  In1 : Inport  Port=2
  Enable : EnablePort
  CAN Transmit1 : arduinolib/CAN Transmit  inputDataType=CAN Msg  BlockingMode_=off  BlockTimeout_=1  outputStatus=off  identifierType=Extended (29-bit identifier)  messageId=position_setpoint  msgLength=4  remoteFrame=off
  Cast To Double1 : DataTypeConversion  OutDataTypeStr=single  SaturateOnIntegerOverflow=off  RndMeth=Floor
  Cast To Double2 : DataTypeConversion  OutDataTypeStr=single  SaturateOnIntegerOverflow=off  RndMeth=Floor
  Give position command : canmsglib/CAN Pack  MsgList=(none)  MsgName=CAN Msg  MsgIDType=Extended (29-bit identifier)  MsgIdentifier=2097174  MsgLength=4  Remote=off  ApplyMinMax=off  BusOutput=on  SignalInfo={ 'position', '0', '32', 'LE', 'single', 'Standard', '0', '1', '0', '-Inf', 'Inf' }
      settings: LibrarySourceBlock=embeddedtargetslib/Host Communication/CAN Pack  DataFormat=manually specified signals
  N-Sample Switch : dspswit3/N-Sample Switch  N=5  reset=off  TriggerType=Rising edge  Ts=1/100
  Position mode : arduinolib/CAN Transmit  inputDataType=Raw data  BlockingMode_=off  BlockTimeout_=1  outputStatus=off  identifierType=Extended (29-bit identifier)  messageId=2097193  msgLength=0  remoteFrame=off
  wires:
  Give position command/1 -> CAN Transmit1/1
  N-Sample Switch/1 -> Give position command/1
  Cast To Double1/1 -> N-Sample Switch/2
  " "/1 -> Cast To Double2/1
  In1/1 -> Cast To Double1/1
  Cast To Double2/1 -> N-Sample Switch/1

== system BuildFlexionExtension2024a/TinyMovr Motor 1/Transmit Velocity/Subsystem ==
  Enable : EnablePort
  Velocity mode : arduinolib/CAN Transmit  inputDataType=Raw data  BlockingMode_=off  BlockTimeout_=1  outputStatus=off  identifierType=Extended (29-bit identifier)  messageId=2097194  msgLength=0  remoteFrame=off

== system BuildFlexionExtension2024a/TinyMovr Motor 1/Transmit Velocity/Subsystem1 ==
  Velocity : Inport  Unit=rad/s
  Enable : EnablePort
  CAN Transmit2 : arduinolib/CAN Transmit  inputDataType=CAN Msg  BlockingMode_=off  BlockTimeout_=1  outputStatus=off  identifierType=Extended (29-bit identifier)  messageId=2097173  msgLength=0  remoteFrame=off
  Cast To Double3 : DataTypeConversion  OutDataTypeStr=single  SaturateOnIntegerOverflow=off  RndMeth=Floor
  Cast To Double4 : DataTypeConversion  OutDataTypeStr=single  SaturateOnIntegerOverflow=off  RndMeth=Floor
  Constant : Constant  Value=0
  Give velocity command : canmsglib/CAN Pack  MsgList=(none)  MsgName=CAN Msg  MsgIDType=Extended (29-bit identifier)  MsgIdentifier=2097176  MsgLength=4  Remote=off  ApplyMinMax=off  BusOutput=on  SignalInfo={ 'velocity', '0', '32', 'LE', 'single', 'Standard', '0', '1', '0', '-Inf', 'Inf' }
      settings: LibrarySourceBlock=embeddedtargetslib/Host Communication/CAN Pack  DataFormat=manually specified signals
  N-Sample Switch1 : dspswit3/N-Sample Switch  N=5  reset=off  TriggerType=Rising edge  Ts=1/100
  Velocity mode : arduinolib/CAN Transmit  inputDataType=Raw data  BlockingMode_=off  BlockTimeout_=1  outputStatus=off  identifierType=Extended (29-bit identifier)  messageId=2097194  msgLength=0  remoteFrame=off
  wires:
  Cast To Double4/1 -> N-Sample Switch1/1
  Velocity/1 -> Cast To Double3/1
  Constant/1 -> Cast To Double4/1
  N-Sample Switch1/1 -> Give velocity command/1
  Cast To Double3/1 -> N-Sample Switch1/2
  Give velocity command/1 -> CAN Transmit2/1

== system BuildFlexionExtension2024a/TinyMovr Motor 2/Transmit Position/Subsystem ==
  Enable : EnablePort
  Byte Unpack : etargetslib/Byte Unpack  dimensions={[1]}  datatypes={'single'}  byteAlign=1
      settings: LibrarySourceBlock=embeddedtargetslib/Host Communication/Byte Unpack
  CAN Receive : arduinolib/CAN Receive  outputDataType=Raw data  identifierType=Extended (29-bit identifier)  messageId=10485813  msgLength=4  SampleTime=1/FSset  outputError=off  outputRemote=off
  CAN Transmit3 : arduinolib/CAN Transmit  inputDataType=Raw data  BlockingMode_=off  BlockTimeout_=1  outputStatus=off  identifierType=Extended (29-bit identifier)  messageId=10485813  msgLength=0  remoteFrame=on
  Terminator : Terminator
  Out1 : Outport
  wires:
  CAN Receive/2 -> Terminator/1
  CAN Receive/1 -> Byte Unpack/1
  Byte Unpack/1 -> Out1/1

== system BuildFlexionExtension2024a/TinyMovr Motor 2/Transmit Position/Subsystem1 ==
  " " : Inport
  In1 : Inport  Port=2
  Enable : EnablePort
  CAN Transmit2 : arduinolib/CAN Transmit  inputDataType=CAN Msg  BlockingMode_=off  BlockTimeout_=1  outputStatus=off  identifierType=Extended (29-bit identifier)  messageId=position_setpoint  msgLength=4  remoteFrame=off
  Cast To Double1 : DataTypeConversion  OutDataTypeStr=single  SaturateOnIntegerOverflow=off  RndMeth=Floor
  Cast To Double2 : DataTypeConversion  OutDataTypeStr=single  SaturateOnIntegerOverflow=off  RndMeth=Floor
  Give position command : canmsglib/CAN Pack  MsgList=(none)  MsgName=CAN Msg  MsgIDType=Extended (29-bit identifier)  MsgIdentifier=10485779  MsgLength=4  Remote=off  ApplyMinMax=off  BusOutput=on  SignalInfo={ 'position', '0', '32', 'LE', 'single', 'Standard', '0', '1', '0', '-Inf', 'Inf' }
      settings: LibrarySourceBlock=embeddedtargetslib/Host Communication/CAN Pack  DataFormat=manually specified signals
  N-Sample Switch : dspswit3/N-Sample Switch  N=5  reset=off  TriggerType=Rising edge  Ts=1/FSset
  Position mode : arduinolib/CAN Transmit  inputDataType=Raw data  BlockingMode_=off  BlockTimeout_=1  outputStatus=off  identifierType=Extended (29-bit identifier)  messageId=10485798  msgLength=0  remoteFrame=off
  wires:
  Give position command/1 -> CAN Transmit2/1
  N-Sample Switch/1 -> Give position command/1
  Cast To Double1/1 -> N-Sample Switch/2
  " "/1 -> Cast To Double2/1
  In1/1 -> Cast To Double1/1
  Cast To Double2/1 -> N-Sample Switch/1

== system BuildFlexionExtension2024a/TinyMovr Motor 2/Transmit Position/Subsystem2 ==
  Enable : EnablePort
  Byte Unpack : etargetslib/Byte Unpack  dimensions={[1]}  datatypes={'single'}  byteAlign=1
      settings: LibrarySourceBlock=embeddedtargetslib/Host Communication/Byte Unpack
  CAN Receive : arduinolib/CAN Receive  outputDataType=Raw data  identifierType=Extended (29-bit identifier)  messageId=4194345  msgLength=4  SampleTime=1/100  outputError=off  outputRemote=off
  CAN Transmit3 : arduinolib/CAN Transmit  inputDataType=Raw data  BlockingMode_=off  BlockTimeout_=1  outputStatus=off  identifierType=Extended (29-bit identifier)  messageId=2097207  msgLength=0  remoteFrame=on
  Terminator : Terminator
  Out1 : Outport
  wires:
  CAN Receive/2 -> Terminator/1
  CAN Receive/1 -> Byte Unpack/1
  Byte Unpack/1 -> Out1/1

== system BuildFlexionExtension2024a/TinyMovr Motor 2/Transmit Position/Subsystem3 ==
  " " : Inport
  In1 : Inport  Port=2
  Enable : EnablePort
  CAN Transmit1 : arduinolib/CAN Transmit  inputDataType=CAN Msg  BlockingMode_=off  BlockTimeout_=1  outputStatus=off  identifierType=Extended (29-bit identifier)  messageId=position_setpoint  msgLength=4  remoteFrame=off
  Cast To Double1 : DataTypeConversion  OutDataTypeStr=single  SaturateOnIntegerOverflow=off  RndMeth=Floor
  Cast To Double2 : DataTypeConversion  OutDataTypeStr=single  SaturateOnIntegerOverflow=off  RndMeth=Floor
  Give position command : canmsglib/CAN Pack  MsgList=(none)  MsgName=CAN Msg  MsgIDType=Extended (29-bit identifier)  MsgIdentifier=4194326  MsgLength=4  Remote=off  ApplyMinMax=off  BusOutput=on  SignalInfo={ 'position', '0', '32', 'LE', 'single', 'Standard', '0', '1', '0', '-Inf', 'Inf' }
      settings: DataFormat=manually specified signals
  N-Sample Switch : dspswit3/N-Sample Switch  N=5  reset=off  TriggerType=Rising edge  Ts=1/100
  Position mode : arduinolib/CAN Transmit  inputDataType=Raw data  BlockingMode_=off  BlockTimeout_=1  outputStatus=off  identifierType=Extended (29-bit identifier)  messageId=4194345  msgLength=0  remoteFrame=off
  wires:
  Give position command/1 -> CAN Transmit1/1
  N-Sample Switch/1 -> Give position command/1
  Cast To Double1/1 -> N-Sample Switch/2
  " "/1 -> Cast To Double2/1
  In1/1 -> Cast To Double1/1
  Cast To Double2/1 -> N-Sample Switch/1

== system BuildFlexionExtension2024a/TinyMovr Motor 2/Transmit Velocity/Subsystem ==
  Enable : EnablePort
  Velocity mode : arduinolib/CAN Transmit  inputDataType=Raw data  BlockingMode_=off  BlockTimeout_=1  outputStatus=off  identifierType=Extended (29-bit identifier)  messageId=2097194  msgLength=0  remoteFrame=off

== system BuildFlexionExtension2024a/TinyMovr Motor 2/Transmit Velocity/Subsystem1 ==
  Velocity : Inport  Unit=rad/s
  Enable : EnablePort
  CAN Transmit2 : arduinolib/CAN Transmit  inputDataType=CAN Msg  BlockingMode_=off  BlockTimeout_=1  outputStatus=off  identifierType=Extended (29-bit identifier)  messageId=2097173  msgLength=0  remoteFrame=off
  Cast To Double3 : DataTypeConversion  OutDataTypeStr=single  SaturateOnIntegerOverflow=off  RndMeth=Floor
  Cast To Double4 : DataTypeConversion  OutDataTypeStr=single  SaturateOnIntegerOverflow=off  RndMeth=Floor
  Constant : Constant  Value=0
  Give velocity command : canmsglib/CAN Pack  MsgList=(none)  MsgName=CAN Msg  MsgIDType=Extended (29-bit identifier)  MsgIdentifier=10485781  MsgLength=4  Remote=off  ApplyMinMax=off  BusOutput=on  SignalInfo={ 'velocity', '0', '32', 'LE', 'single', 'Standard', '0', '1', '0', '-Inf', 'Inf' }
      settings: LibrarySourceBlock=embeddedtargetslib/Host Communication/CAN Pack  DataFormat=manually specified signals
  N-Sample Switch1 : dspswit3/N-Sample Switch  N=5  reset=off  TriggerType=Rising edge  Ts=1/FSset
  Velocity mode : arduinolib/CAN Transmit  inputDataType=Raw data  BlockingMode_=off  BlockTimeout_=1  outputStatus=off  identifierType=Extended (29-bit identifier)  messageId=10485799  msgLength=0  remoteFrame=off
  wires:
  Cast To Double4/1 -> N-Sample Switch1/1
  Velocity/1 -> Cast To Double3/1
  Constant/1 -> Cast To Double4/1
  N-Sample Switch1/1 -> Give velocity command/1
  Cast To Double3/1 -> N-Sample Switch1/2
  Give velocity command/1 -> CAN Transmit2/1

== matlab function BuildFlexionExtension2024a/IMU/MATLAB Function2 ==
  data: y input; x_hat output
function x_hat = kalman_hip(y)
% y: measured angle (scalar)
% x_hat: [theta_hat; theta_dot_hat]

persistent A C Q R P x
persistent initialized

Ts = 0.01; % sample time

if isempty(initialized)
    A = [1 Ts; 0 1];
    C = [1 0];

    % Tune these:
    Q = [1e-6      0;
        0      5e-3];   % more process noise on velocity state
    R = 4e-4;            % measurement noise variance (rad^2)

    P = eye(2);        % initial covariance
    x = [0; 0];        % initial state estimate
    initialized = true;
end

% Prediction
x_pred = A * x;
P_pred = A * P * A' + Q;

% Innovation
y_pred = C * x_pred;
e = y - y_pred;  % innovation

S = C * P_pred * C' + R;
K = P_pred * C' / S;  % Kalman gain (2x1)

% Update
x = x_pred + K * e;
P = (eye(2) - K * C) * P_pred;

x_hat = x;

== matlab function BuildFlexionExtension2024a/IMU/MATLAB Function1 ==
  data: y input; x_hat output
function x_hat = kalman_hip(y)
% y: measured angle (scalar)
% x_hat: [theta_hat; theta_dot_hat]

persistent A C Q R P x
persistent initialized

Ts = 0.01; % sample time

if isempty(initialized)
    A = [1 Ts; 0 1];
    C = [1 0];

    % Tune these:
    Q = [1e-6      0;
        0      5e-3];   % more process noise on velocity state
    R = 4e-4;            % measurement noise variance (rad^2)

    P = eye(2);        % initial covariance
    x = [0; 0];        % initial state estimate
    initialized = true;
end

% Prediction
x_pred = A * x;
P_pred = A * P * A' + Q;

% Innovation
y_pred = C * x_pred;
e = y - y_pred;  % innovation

S = C * P_pred * C' + R;
K = P_pred * C' / S;  % Kalman gain (2x1)

% Update
x = x_pred + K * e;
P = (eye(2) - K * C) * P_pred;

x_hat = x;
